simulink model "sim_ekf_est_motor_4para"  (R2020b)
settings: Solver=ode1  StartTime=0.0  StopTime=100  FixedStep=0.01  RelTol=1e-3
undefined symbols (not defined in the file): DiscIntNeverNeededParam
settings Model: Creator=Admin  LastModifiedBy=ONLY-GOD

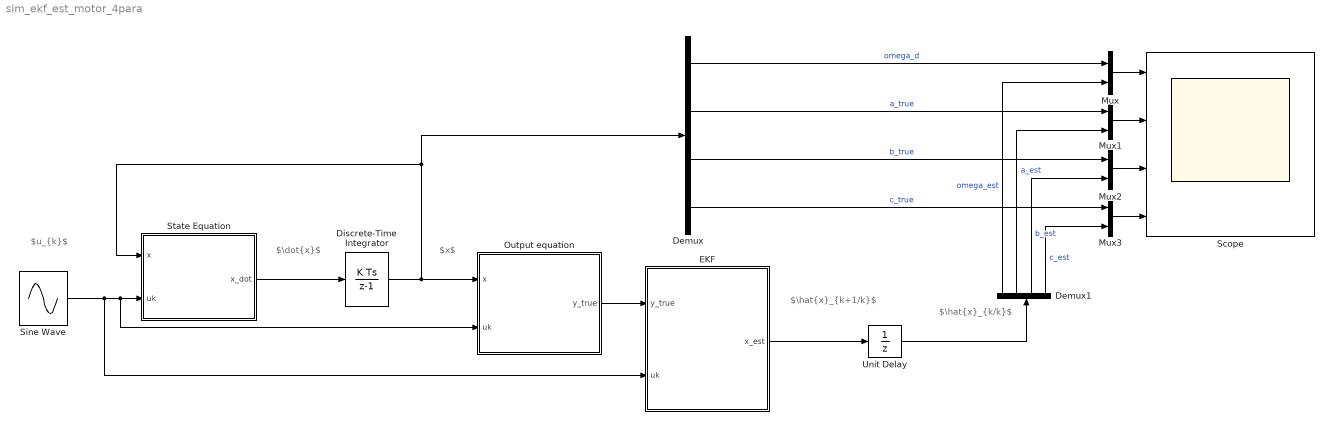
== system sim_ekf_est_motor_4para ==
  note: $\dot{x}$
  note: $x$
  note: $u_{k}$
  note: $\hat{x}_{k+1/k}$
  note: $\hat{x}_{k/k}$
  Demux : Demux
  Demux1 : Demux
  Discrete-Time Integrator : DiscreteIntegrator  InitialCondition=[0;20;40;5]  SampleTime=-1  ICPrevOutput=DiscIntNeverNeededParam  ICPrevScaledInput=DiscIntNeverNeededParam
  EKF : MATLAB Function  TreatAsAtomicUnit=on
  Mux{,1..3} (4 alike) : Mux  Inputs=2
  Output equation : MATLAB Function  TreatAsAtomicUnit=on
  Scope : Scope  NumInputPorts=4
  Sine Wave : Sin  Amplitude=20  Frequency=2*pi*0.1  SampleTime=0
  State Equation : MATLAB Function  TreatAsAtomicUnit=on
  Unit Delay : UnitDelay  InitialCondition=[0;0;0;0]  SampleTime=-1  HasFrameUpgradeWarning=on
  wires:
  State Equation/1(x_dot) -> Discrete-Time Integrator/1
  Discrete-Time Integrator/1 -> State Equation/1(x), Demux/1, Output equation/1(x)
  Output equation/1(y_true) -> EKF/1(y_true)
  EKF/1(x_est) -> Unit Delay/1
  Unit Delay/1 -> Demux1/1
  Demux/1 -> Mux/1  "omega_d"
  Demux1/1 -> Mux/2  "omega_est"
  Mux/1 -> Scope/1
  Demux/2 -> Mux1/1  "a_true"
  Demux1/2 -> Mux1/2  "a_est"
  Demux/3 -> Mux2/1  "b_true"
  Demux1/3 -> Mux2/2  "b_est"
  Mux1/1 -> Scope/2
  Mux2/1 -> Scope/3
  Sine Wave/1 -> EKF/2(uk), Output equation/2(uk), State Equation/2(uk)
  Demux/4 -> Mux3/1  "c_true"
  Demux1/4 -> Mux3/2  "c_est"
  Mux3/1 -> Scope/4

== matlab function sim_ekf_est_motor_4para/EKF ==
  settings: updateMethod=DISCRETE
  data: y_true input; uk input; x_est output
function x_est = ekf(y_true, uk)
Ts = 0.01;
persistent x_est_p P Qd_est R_est Qc_est;
if isempty(x_est_p)
    x_est_p = [0;0;0;0];
    P       = 1e-4*diag([10,1,30,10]);
    Qc_est  = 1e-4*diag([1,10,100,10]);
    Qd_est  = Ts*Qc_est;
    R_est   = 0.001;
end
c  = [1 0 0 0];
D  = 0;
Ck = c;
Dk = D;

%Comput Kalman Gain and update predicted value
Wk    = P*Ck'/(Ck*P*Ck'+R_est);
y_est = Ck*x_est_p+Dk*uk;
x     = x_est_p+Wk.*(y_true-y_est);

%Compute prediction at next time step
x_est = x+Ts*[-x(2)*x(1)+uk*x(3)-x(4)*sign(x(1));
                          0;
                          0;
                          0];

%Update error covariance matrices
P = P-Wk*Ck*P;

%Define Ak
Ak      = eye(4)+Ts*[-x(2) -x(1) uk -sign(x(1));
                 0     0    0      0;
                 0     0    0      0;
                 0     0    0      0];
P       = Ak*P*Ak'+Qd_est;
x_est_p = x_est;

== matlab function sim_ekf_est_motor_4para/State Equation ==
  settings: updateMethod=DISCRETE
  data: x input; uk input; x_dot output
function x_dot = state_eq(x,uk)
x_dot = [0;0;0;0];
x_dot(1) = -x(1)*x(2)+x(3)*uk+sqrt(0.02)-x(4)*sign(x(1))*sqrt(0.01)*randn;
x_dot(2) = 0;
x_dot(3) = 0;
x_dot(4) = 0;

== matlab function sim_ekf_est_motor_4para/Output equation ==
  settings: updateMethod=DISCRETE
  data: x input; uk input; y_true output
function y_true = output_eq(x,uk)
C = [1 0 0 0];
D = 0;
y_true = C*x+D*uk+sqrt(0.02)*randn;
